simulink model "PMSM_traditional_SMO_PLL_Leon"  (R2024b)
settings: Solver=FixedStepAuto  StartTime=0.0  StopTime=0.5  FixedStep=1e-6  RelTol=1e-4  EnableMultiTasking=on
PreLoadFcn:
  | flux =0.0037
  | Ld =1.2050e-04
  | Lq =1.8000e-04
  | Pn =4
  | R =0.0830
  | Ts =5.0000e-05
undefined symbols (not defined in the file): DiscIntNeverNeededParam
libraries: mcbcontrolslib x3, simulink x2, powerlib_extras x2, spsDCVoltageSourceLib x1, spsPermanentMagnetSynchronousMachineLib x1, spsUniversalBridgeLib x1, spspowerguiLib x1
settings Model: LastModifiedBy=SESA504213
settings SolverCC: ZeroCrossControl=DisableAll  AlgebraicLoopSolver=TrustRegion  AutoInsertRateTranBlk=on
settings DataIOCC: LimitDataPoints=on  SaveFormat=Array  SignalLoggingSaveFormat=ModelDataLogs  ReturnWorkspaceOutputs=off
settings OptimizationCC: ReuseModelBlockBuffer=off  ExpressionDepthLimit=2147483647  InitFltsAndDblsToZero=on  LifeSpan=inf
settings DebuggingCC: UnderspecifiedInitializationDetection=Classic  MergeDetectMultiDrivingBlocksExec=none  SolverPrmCheckMsg=warning  FcnCallInpInsideContextMsg=warning  UnconnectedInputMsg=warning  UnconnectedOutputMsg=warning  UnconnectedLineMsg=warning  StateNameClashWarn=warning  SFUnexpectedBacktrackingDiag=warning  SFNoUnconditionalDefaultTransitionDiag=warning  SFExecutionAtInitializationDiag=none  ArithmeticOperatorsInVariantConditions=warning
settings HardwareCC: ProdBitPerPointer=32  ProdBitPerSizeT=32  ProdBitPerPtrDiffT=32  ProdLargestAtomicFloat=None  ProdIntDivRoundTo=Undefined  ProdEndianess=Unspecified  ProdWordSize=32  ProdHWDeviceType=32-bit Generic
settings ModelReferenceCC: EnableRefExpFcnMdlSchedulingChecks=on  PropagateSignalLabelsOutOfModel=off
settings SFSimCC: SimUseLocalCustomCode=off  CustomCodeUndefinedFunction=UseInterfaceOnly
settings RTWCC: RTWUseLocalCustomCode=off  GPUComputeCapability=3.5  DLArmComputeVersion=19.05
settings CodeAppCC: StateflowObjectComments=on
settings GRTTargetCC: TargetLangStandard=C89/C90 (ANSI)  CombineOutputUpdateFcns=off  GRTInterface=on
settings ConfigComp: CovMetricSettings=dw  CovSaveCumulativeToWorkspaceVar=on  CovSaveSingleToWorkspaceVar=on  CovExternalEMLEnable=off  CovSFcnEnable=off
settings SimscapeCC: SimscapeNormalizeSystem=off

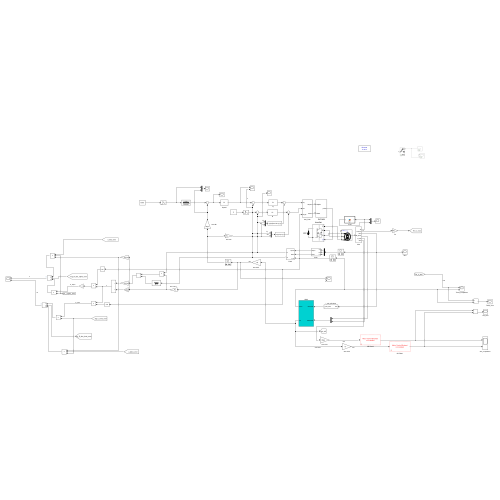
[thumbnail: Simulink's stored preview of the top-level diagram]
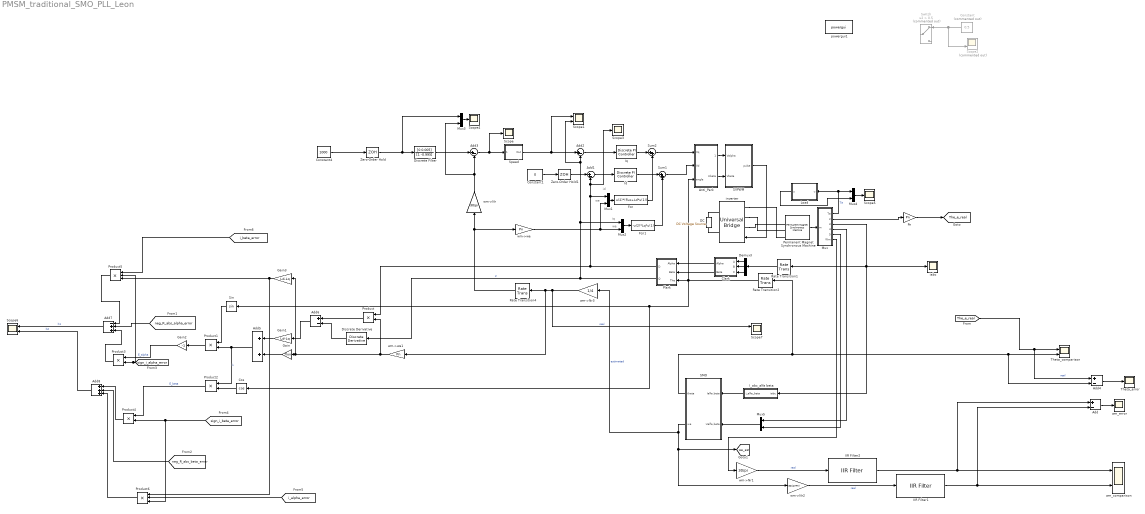
== system PMSM_traditional_SMO_PLL_Leon ==
  note: iq
  note: we
  note: we
  note: id
  Add : Sum  Inputs=+-
  Add1 : Sum  Inputs=|+-
  Add2 : Sum  Inputs=|+-
  Add3 : Sum  Inputs=|+-
  Add4 : Sum  Inputs=+-
  Add5 : Sum
  Add6 : Sum  Inputs=+-
  Add7 : Sum  Inputs=-++
  Add8 : Sum  Inputs=+++
  Anti_Park : Subsystem
  Clark : Subsystem
  Constant : Constant  Commented=on  Value=0.5
  Constant1 : Constant  Value=0
  Constant4 : Constant  Value=1000
  Cos : Trigonometry  Operator=cos
  DC : spsDCVoltageSourceLib/DC Voltage Source  Amplitude=24  Measurements=None
  Demux3 : Demux  Outputs=3
  Discrete Derivative : simulink/Discrete/Discrete Derivative  gainval=1.0  ICPrevScaledInput=0.0  OutMin=[]  OutMax=[]  OutDataType=fixdt(1, 16)  OutScaling=2^-10  DoSatur=off
  Discrete Filter : DiscreteFilter  Numerator=[0 0.005]  Denominator=[1 -0.995]  InitialStates=0.001
  Fcn : Fcn  Expr=u(2)*(flux+Ld*u(1))
  Fcn1 : Fcn  Expr=-u(2)*Lq*u(1)
  Gain : Gain  Gain=flux
  Gain1 : Gain  Gain=Ld-Lq
  Gain2 : Gain  Gain=-1
  Gain3 : Gain  Gain=Ld-Lq
  IIR Filter1 : mcbcontrolslib/IIR Filter  VariantControl=Low Pass Filter  VariantSelect=Low-pass  Filter_constant=0.0004  advancedSettings=on  Ts=1e-6  cutOff_freq=63.6875
  IIR Filter2 : mcbcontrolslib/IIR Filter  VariantControl=Low Pass Filter  VariantSelect=Low-pass  Filter_constant=0.0004  advancedSettings=on  Ts=1e-6  cutOff_freq=63.6875
  I_abc_alfa beta : Subsystem
  Id : powerlib_extras/Discrete  Control Blocks/Discrete PI Controller  Kp=Ld*4000/2  Ki=R*4000/2  Par_Limits=[24*0.9*sqrt(1/3) -24*0.9*sqrt(1/3)]  Init=0  Ts=Ts
  Iq : powerlib_extras/Discrete  Control Blocks/Discrete PI Controller  Kp=Lq*4000/2  Ki=R*4000/2  Par_Limits=[24*0.9*sqrt(1/3) -24*0.9*sqrt(1/3)]  Init=0  Ts=Ts
  Load : MATLAB Function  TreatAsAtomicUnit=on
  Mux : Subsystem
  Mux{1..5} (5 alike) : Mux  Inputs=2
  Permanent Magnet Synchronous Machine : spsPermanentMagnetSynchronousMachineLib/Permanent Magnet Synchronous Machine  NbPhases=3  FluxDistribution=Sinusoidal  RotorType=Salient-pole  MechanicalLoad=Torque Tm  PresetModel=No  ShowDetailedParameters=on  MeasurementBus=off  Resistance=R  Inductance=0  dqInductances=[Ld,Lq]  La=0.000835  MachineConstant=Flux linkage established by magnets (V.s)  Flux=flux  VoltageCst=2.6844  TorqueCst=0.0222  Flat=0  Mechanical=[1e-5,1e-5,Pn]  PolePairs=4  InitialConditions=[0,0,0,0]  InitialConditions5ph=[0 0 0 0 0 0]  RefAngle=Aligned with phase A axis (original Park)  IterativeDiscreteModel=Trapezoidal non iterative  TsBlock=-1  TsPowergui=0
      settings: AttributesFormatString=\n
  Plark : Subsystem
  Pn : Gain  Gain=Pn
  Product{,1..4} (5 alike) : Product
  Product5 : Product  Inputs=3
  Product6 : Product  Inputs=3
  Rate Transition1 : RateTransition  OutPortSampleTime=Ts
  Rate Transition2 : RateTransition  OutPortSampleTime=Ts
  Rate Transition4 : RateTransition  OutPortSampleTime=Ts
  SMO : Subsystem
  SVPWM : Subsystem
  Scope{,3..5} (4 alike) : Scope
  Scope1 : Scope  NumInputPorts=2
  Scope2 : Scope  Commented=on  NumInputPorts=2
  Scope6 : Scope  NumInputPorts=2
  Scope7 : Scope  NumInputPorts=2
  Sin : Trigonometry
  Speed : Subsystem  AncestorBlock=|  DialogController=POWERSYS.PowerSysDialog  mask(Discrete PI Controller){Kp=0.0453/2, Ki=1.1381/2, Par_Limits=[30 -30], Init=0, Ts=Ts}
      | powerlib_extras/Discrete 
      | Control Blocks/Discrete
      | PI Controller
      mask prompts: Kp "Proportional gain (Kp):"; Ki "Integral gain (Ki):"; Par_Limits "Output limits: [ Upper   Lower ]"; Init "Output initial value:"; Ts "Sample time:"
      mask help: This block implements a discrete PI controller.
      mask init:
      | UpperLimit=Par_Limits(1);
      | LowerLimit=Par_Limits(2);
      | power_initmask();
      mask Help: This block is part of a subset of blocks in the Extras library that does not have documentation associated with it, other than the block mask description.
      mask Display: disp('PI');
  Sum1 : Sum  Inputs=|++
  Sum2 : Sum  Inputs=|++
  Switch : Switch  Commented=on  Criteria=u2 > Threshold  Threshold=0.5  SaturateOnIntegerOverflow=off  InputSameDT=off
  Theta_comparison : Scope  NumInputPorts=2
  Theta_error : Scope
  Zero-Order Hold : ZeroOrderHold  SampleTime=Ts
  Zero-Order Hold1 : ZeroOrderHold  SampleTime=Ts
  iabc : Scope
  inverter : spsUniversalBridgeLib/Universal Bridge  Arms=3  SnubberResistance=100  SnubberCapacitance=1e-5  Device=MOSFET / Diodes  Ron=1e-3  Lon=0  ForwardVoltages="[  0  0  ]"  ForwardVoltage=0  GTOparameters=[ 10e-6 , 20e-6 ]  IGBTparameters=[ 1e-6 , 2e-6 ]  Measurements=None  Measurements_2=None  converterType=Rectifier
  powergui1 : spspowerguiLib/powergui  Priority=1  SimulationMode=Discrete  SampleTime=1e-6  frequency=60  Iterations=50  frequencyindice=0  Pbase=100e6  ErrMax=1e-4  UnitsV=kV  UnitsW=MW  buscounter=0  FunctionMessages=off  echomessages=off  EnableUseOfTLC=off  CurrentSourceSwitches=off  DisableSnubberDevices=off  DisableRonSwitches=off  DisableVfSwitches=off  DisplayEquations=off  AutomaticDiscreteSolvers=off  SolverType=Tustin/Backward Euler (TBE)  Interpol=off  ExternalGateDelay=off  methode=off  Ts=100  x0status=blocks  SPID=on  SwTol=0  HookPort=off  NonlinearTolerance=1e-4  nMaxIteration=100  ContinueOnMaxIteration=off  RestoreLinks=warning  ResistiveCurrentMeasurement=off  Frange=[0:2:500]  Ylog=off  Xlog=on  ShowGrid=off  save=off  variable=ZData  structure=0  ZoomFFT=off  StartTime=0.0  cycles=1  DisplayStyle=1  fundamental=60  FreqAxis=off  MaxFrequency=1000  frequencyindicesteady=1  RmsSteady=1  display=off
  wm->Nr : Gain  Gain=30/pi
  wm->Nr1 : Gain  Gain=30/pi
  wm->Nr2 : Gain  Gain=30/(pi*Pn)
  wm->Nr3 : Gain  Gain=1/4
  wm->we : Gain  Gain=Pn
  wm->we1 : Gain  Gain=Pn
  wm_comparison : Scope  NumInputPorts=2
  wm_error : Scope
  tag scope: The_e_real=global, we_est=global
  wires:
  Permanent Magnet Synchronous Machine/1 -> Mux/1(m)
  Add3/1 -> Speed/1(Error), Scope/1
  Fcn/1 -> Sum2/2
  Fcn1/1 -> Sum1/2
  Add1/1 -> Id/1
  wm->Nr/1 -> Mux3/2, Add3/2
  Id/1 -> Sum1/1
  wm->we/1 -> Mux2/2, Mux1/2
  Mux1/1 -> Fcn/1
  Mux2/1 -> Fcn1/1
  Add2/1 -> Iq/1
  Iq/1 -> Sum2/1
  Sum2/1 -> Anti_Park/1(Vq)
  Sum1/1 -> Anti_Park/2(Vd)
  Mux/2(Thetam) -> Pn/1
  SVPWM/1(pulse) -> inverter/1
  Anti_Park/1(Ualpha) -> SVPWM/1(Valpha)
  Anti_Park/2(Ubeta) -> SVPWM/2(Vbeta)
  Clark/1(Alpha) -> Plark/1(Alpha)
  Demux3/1 -> Clark/1(A)
  Demux3/2 -> Clark/2(B)
  Demux3/3 -> Clark/3(C)
  Clark/2(Beta) -> Plark/2(Beta)
  Plark/2(Q) -> Discrete Derivative/1, Mux2/1, Scope1/2, Add2/2  "2"
  Constant/1 -> Scope2/2, Switch/1
  Speed/1(Out) -> Scope1/1, Add2/1
  Mux/3(Iabc) -> I_abc_alfa beta/1(iabc), Rate Transition1/1, iabc/1
  Pn/1 -> [The_e_real]
  Plark/1(D) -> Product/1, Mux1/1, Scope3/1, Add1/2
  Rate Transition4/1 -> wm->Nr/1, wm->we/1
  Constant4/1 -> Zero-Order Hold/1
  Constant1/1 -> Zero-Order Hold1/1
  Zero-Order Hold1/1 -> Add1/1
  Rate Transition1/1 -> Demux3/1
  Rate Transition2/1 -> Cos/1, Sin/1, Anti_Park/3(angle), Plark/3(The)
  Zero-Order Hold/1 -> Mux3/1, Discrete Filter/1
  Discrete Filter/1 -> Add3/1
  Mux3/1 -> Scope4/1
  Load/1(y) -> Mux4/2
  Mux/1(Te) -> Mux4/1, Load/1(u)  "Te"
  Mux4/1 -> Scope5/1
  I_abc_alfa beta/1(i_alfa_beta) -> SMO/1(Ialfa,beta)
  Mux5/1 -> SMO/2(Ualfa,beta)
  SMO/1(theta) -> Rate Transition2/1, Add4/2, Theta_comparison/2
  wm->Nr1/1 -> IIR Filter2/1  "real"
  SMO/2(we) -> wm->Nr3/1, wm->Nr2/1, [we_est]  "estimated"
  [The_e_real] -> Add4/1, Theta_comparison/1  "real"
  Add/1 -> wm_error/1
  Add4/1 -> Theta_error/1
  Mux/4(u_alpha) -> Mux5/1
  Mux/5(u_beta) -> Mux5/2
  wm->Nr2/1 -> IIR Filter1/1  "real"
  wm->we1/1 -> Gain3/1, Gain/1, Product/2
  Gain/1 -> Add5/2
  Gain1/1 -> Add5/1
  Product/1 -> Add6/1
  Discrete Derivative/1 -> Add6/2
  Add6/1 -> Gain1/1
  Add5/1 -> Product2/1, Product1/2  "k"
  Sin/1 -> Product1/1
  Product1/1 -> Gain2/1
  Gain2/1 -> Product3/1  "E_alpha"
  Cos/1 -> Product2/2
  Product2/1 -> Product4/1  "E_beta"
  [neg_R_abs_beta_error] -> Add8/2
  Add7/1 -> Scope6/1  "h1"
  Add8/1 -> Scope6/2  "h2"
  [sign_i_alpha_error] -> Product3/2, Product5/2
  Product4/1 -> Add8/1
  [sign_i_beta_error] -> Product6/3, Product4/2
  Product3/1 -> Add7/3
  [neg_R_abs_alpha_error] -> Add7/2
  Gain3/1 -> Product5/3, Product6/1
  [i_beta_error] -> Product5/1
  Product5/1 -> Add7/1
  Product6/1 -> Add8/3
  [i_alpha_error] -> Product6/2
  IIR Filter1/1 -> Add/2, wm_comparison/2
  IIR Filter2/1 -> Add/1, wm_comparison/1
  wm->Nr3/1 -> Scope7/1, wm->we1/1, Rate Transition4/1  "real"
  Mux/6(Wm) -> wm->Nr1/1
  connections:
  DC/RConn1 -- inverter/RConn1
  DC/LConn1 -- inverter/RConn2
  inverter/LConn1 -- Permanent Magnet Synchronous Machine/LConn1
  inverter/LConn2 -- Permanent Magnet Synchronous Machine/LConn2
  inverter/LConn3 -- Permanent Magnet Synchronous Machine/LConn3

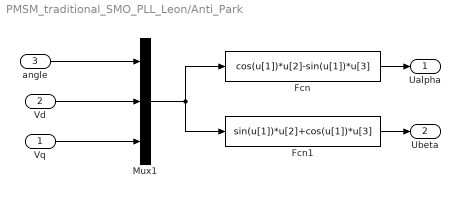
== system PMSM_traditional_SMO_PLL_Leon/Anti_Park ==
  Vq : Inport
  Vd : Inport  Port=2
  angle : Inport  Port=3
  Fcn : Fcn  Expr=cos(u[1])*u[2]-sin(u[1])*u[3]
  Fcn1 : Fcn  Expr=sin(u[1])*u[2]+cos(u[1])*u[3]
  Mux1 : Mux  Inputs=3
  Ualpha : Outport
  Ubeta : Outport  Port=2
  wires:
  Fcn1/1 -> Ubeta/1
  Fcn/1 -> Ualpha/1
  Mux1/1 -> Fcn/1, Fcn1/1
  Vd/1 -> Mux1/2
  Vq/1 -> Mux1/3
  angle/1 -> Mux1/1

== system PMSM_traditional_SMO_PLL_Leon/Clark ==
  A : Inport
  B : Inport  Port=2
  C : Inport  Port=3
  Mux : Mux  Inputs=3
  alpha : Fcn  Expr=(u(1)-0.5*(u(2)+u(3)))*2/3
  beta : Fcn  Expr=sqrt(3)/2*(u(2)-u(3))*2/3
  Alpha : Outport
  Beta : Outport  Port=2
  wires:
  alpha/1 -> Alpha/1
  B/1 -> Mux/2
  C/1 -> Mux/3
  A/1 -> Mux/1
  Mux/1 -> beta/1, alpha/1
  beta/1 -> Beta/1

== system PMSM_traditional_SMO_PLL_Leon/I_abc_alfa beta ==
  iabc : Inport
  Fcn : Fcn  Expr=(2*u(1)-u(2)-u(3))/3
  Fcn1 : Fcn  Expr=(u(2)-u(3))/(3^(1/2))
  Mux2 : Mux  Inputs=2
  i_alfa_beta : Outport
  wires:
  iabc/1 -> Fcn/1, Fcn1/1
  Mux2/1 -> i_alfa_beta/1
  Fcn/1 -> Mux2/1
  Fcn1/1 -> Mux2/2

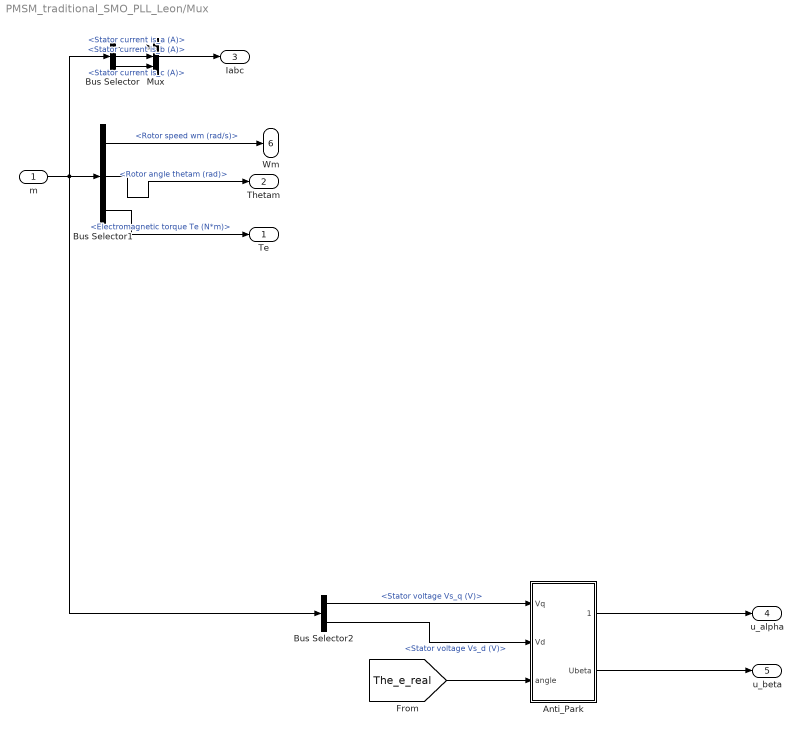
== system PMSM_traditional_SMO_PLL_Leon/Mux ==
  m : Inport
  Anti_Park : Subsystem
  Bus Selector : BusSelector  OutputSignals=Stator current is_a (A),Stator current is_b (A),Stator current is_c (A)
  Bus Selector1 : BusSelector  OutputSignals=Rotor speed wm (rad/s),Rotor angle thetam (rad),Electromagnetic torque Te (N*m)
  Bus Selector2 : BusSelector  OutputSignals=Stator voltage Vs_q (V),Stator voltage Vs_d (V)
  Mux : Mux  Inputs=3
  Te : Outport
  Thetam : Outport  Port=2
  Iabc : Outport  Port=3
  u_alpha : Outport  Port=4
  u_beta : Outport  Port=5
  Wm : Outport  Port=6
  wires:
  Bus Selector1/1 -> Wm/1  "<Rotor speed wm (rad/s)>"
  Bus Selector1/2 -> Thetam/1  "<Rotor angle thetam (rad)>"
  Bus Selector1/3 -> Te/1  "<Electromagnetic torque Te (N*m)>"
  m/1 -> Bus Selector2/1, Bus Selector/1, Bus Selector1/1
  Bus Selector/2 -> Mux/2  "<Stator current is_b (A)>"
  Bus Selector/3 -> Mux/3  "<Stator current is_c (A)>"
  Bus Selector/1 -> Mux/1  "<Stator current is_a (A)>"
  Mux/1 -> Iabc/1
  Bus Selector2/2 -> Anti_Park/2(Vd)  "<Stator voltage Vs_d (V)>"
  Bus Selector2/1 -> Anti_Park/1(Vq)  "<Stator voltage Vs_q (V)>"
  Anti_Park/1(Ualpha) -> u_alpha/1
  [The_e_real] -> Anti_Park/3(angle)
  Anti_Park/2(Ubeta) -> u_beta/1

== system PMSM_traditional_SMO_PLL_Leon/Plark ==
  Alpha : Inport
  Beta : Inport  Port=2
  The : Inport  Port=3
  Mux : Mux  Inputs=3
  d : Fcn  Expr=u(1)*cos(u(3))+u(2)*sin(u(3))
  q : Fcn  Expr=-u(1)*sin(u(3))+u(2)*cos(u(3))
  D : Outport
  Q : Outport  Port=2
  wires:
  d/1 -> D/1
  Beta/1 -> Mux/2
  Alpha/1 -> Mux/1
  Mux/1 -> q/1, d/1
  q/1 -> Q/1
  The/1 -> Mux/3

== system PMSM_traditional_SMO_PLL_Leon/SMO ==
  Ialfa,beta : Inport
  Ualfa,beta : Inport  Port=2
  PLL : Subsystem
  SMO : Subsystem
  theta : Outport
  we : Outport  Port=2
  wires:
  Ualfa,beta/1 -> SMO/1(Ualfa,beta)
  Ialfa,beta/1 -> SMO/2(Ialfa,beta)
  SMO/1(Ealpha^) -> PLL/1(e_alpha_est)
  SMO/2(Ebeta^) -> PLL/2(e_beta_est)
  PLL/1(theta_est) -> theta/1
  PLL/2(we_est) -> we/1

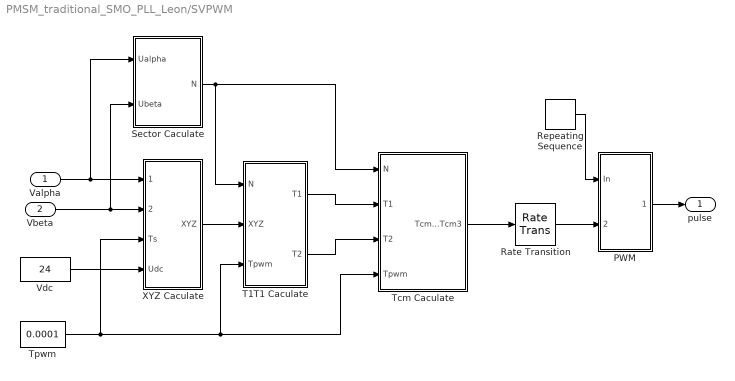
== system PMSM_traditional_SMO_PLL_Leon/SVPWM ==
  Valpha : Inport
  Vbeta : Inport  Port=2
  PWM : Subsystem
  Rate Transition : RateTransition  OutPortSampleTime=1e-6
  Repeating Sequence : simulink/Sources/Repeating Sequence  rep_seq_t=[0 0.00005 0.0001]  rep_seq_y=[0 0.00005 0]
  Sector Caculate : Subsystem
  T1T1 Caculate : Subsystem
  Tcm Caculate : Subsystem
  Tpwm : Constant  Value=0.0001
  Vdc : Constant  Value=24
  XYZ Caculate : Subsystem
  pulse : Outport
  wires:
  PWM/1(PWM) -> pulse/1
  Repeating Sequence/1 -> PWM/1(In)
  Vbeta/1 -> XYZ Caculate/2(Ubeta), Sector Caculate/2(Ubeta)
  T1T1 Caculate/1(T1) -> Tcm Caculate/2(T1)
  Valpha/1 -> XYZ Caculate/1(Ualpha), Sector Caculate/1(Ualpha)
  T1T1 Caculate/2(T2) -> Tcm Caculate/3(T2)
  Sector Caculate/1("N ") -> Tcm Caculate/1(N), T1T1 Caculate/1(N)
  XYZ Caculate/1(XYZ) -> T1T1 Caculate/2(XYZ)
  Tpwm/1 -> XYZ Caculate/3(Ts), Tcm Caculate/4(Tpwm), T1T1 Caculate/3(Tpwm)
  Vdc/1 -> XYZ Caculate/4(Udc)
  Tcm Caculate/1(Tcm1 Tcm2 Tcm3) -> Rate Transition/1
  Rate Transition/1 -> PWM/2(Tcm123)

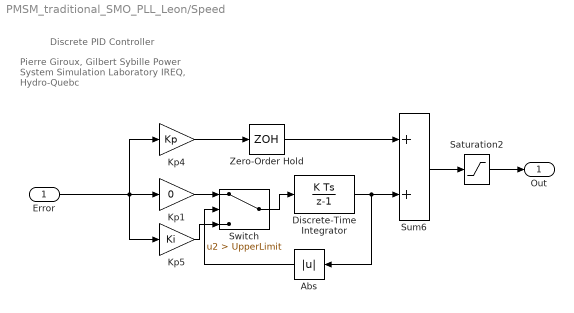
== system PMSM_traditional_SMO_PLL_Leon/Speed ==
  note: Discrete PID Controller
  note: Pierre Giroux, Gilbert Sybille
      | Power System Simulation Laboratory
      | IREQ, Hydro-Quebc
  Error : Inport  SampleTime=Ts
  Abs : Abs  SaturateOnIntegerOverflow=off
  Discrete-Time Integrator : DiscreteIntegrator  InitialCondition=Init  SampleTime=Ts  LimitOutput=on  UpperSaturationLimit=UpperLimit  LowerSaturationLimit=LowerLimit  ICPrevOutput=DiscIntNeverNeededParam  ICPrevScaledInput=DiscIntNeverNeededParam
  Kp1 : Gain  Gain=0  SaturateOnIntegerOverflow=on  SampleTime=Ts  OutDataTypeStr=Inherit: Same as input  ParamDataTypeStr=Inherit: Same as input
  Kp4 : Gain  Gain=Kp  SaturateOnIntegerOverflow=on  SampleTime=Ts  OutDataTypeStr=Inherit: Same as input  ParamDataTypeStr=Inherit: Same as input
  Kp5 : Gain  Gain=Ki  SaturateOnIntegerOverflow=on  SampleTime=Ts  OutDataTypeStr=Inherit: Same as input  ParamDataTypeStr=Inherit: Same as input
  Saturation2 : Saturate  UpperLimit=UpperLimit  LowerLimit=LowerLimit  SampleTime=Ts
  Sum6 : Sum  InputSameDT=on  SaturateOnIntegerOverflow=on  SampleTime=Ts  OutDataTypeStr=Inherit: Same as first input
  Switch : Switch  Criteria=u2 > Threshold  Threshold=UpperLimit  SaturateOnIntegerOverflow=off  InputSameDT=off
  Zero-Order Hold : ZeroOrderHold  SampleTime=Ts
  Out : Outport  SampleTime=Ts  InitialOutput=0  VectorParamsAs1DForOutWhenUnconnected=off
  wires:
  Zero-Order Hold/1 -> Sum6/1
  Saturation2/1 -> Out/1
  Discrete-Time Integrator/1 -> Abs/1, Sum6/2
  Kp4/1 -> Zero-Order Hold/1
  Sum6/1 -> Saturation2/1
  Error/1 -> Kp4/1, Kp1/1, Kp5/1
  Switch/1 -> Discrete-Time Integrator/1
  Abs/1 -> Switch/2
  Kp5/1 -> Switch/3
  Kp1/1 -> Switch/1

== system PMSM_traditional_SMO_PLL_Leon/Mux/Anti_Park ==
  Vq : Inport
  Vd : Inport  Port=2
  angle : Inport  Port=3
  Fcn : Fcn  Expr=cos(u[1])*u[2]-sin(u[1])*u[3]
  Fcn1 : Fcn  Expr=sin(u[1])*u[2]+cos(u[1])*u[3]
  Mux1 : Mux  Inputs=3
  Ualpha : Outport
  Ubeta : Outport  Port=2
  wires:
  Fcn1/1 -> Ubeta/1
  Fcn/1 -> Ualpha/1
  Mux1/1 -> Fcn/1, Fcn1/1
  Vd/1 -> Mux1/2
  Vq/1 -> Mux1/3
  angle/1 -> Mux1/1

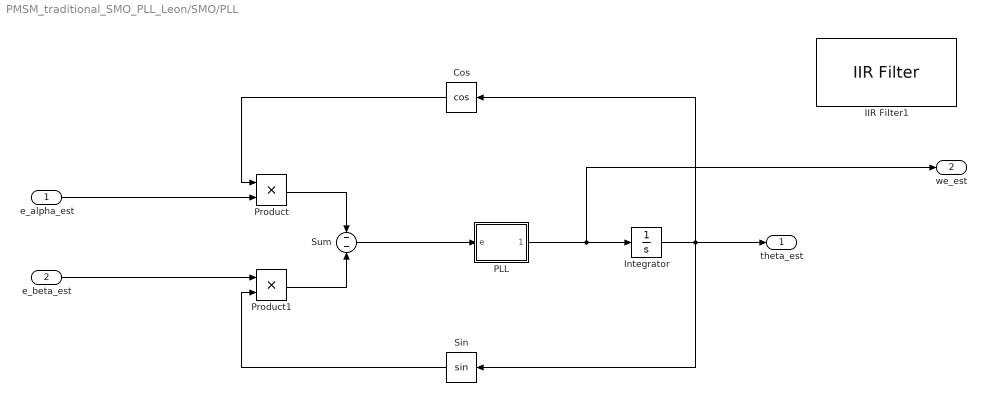
== system PMSM_traditional_SMO_PLL_Leon/SMO/PLL ==
  e_alpha_est : Inport
  e_beta_est : Inport  Port=2
  Cos : Trigonometry  Operator=cos
  IIR Filter1 : mcbcontrolslib/IIR Filter  VariantControl=Low Pass Filter  VariantSelect=Low-pass  Filter_constant=0.0004  advancedSettings=on  Ts=1e-6  cutOff_freq=63.6875
  Integrator : Integrator
  PLL : Subsystem
      mask Display: disp('PI')
  Product : Product
  Product1 : Product
  Sin : Trigonometry
  Sum : Sum  Inputs=--
  theta_est : Outport
  we_est : Outport  Port=2
  wires:
  e_alpha_est/1 -> Product/2
  Cos/1 -> Product/1
  Product/1 -> Sum/1
  e_beta_est/1 -> Product1/1
  Product1/1 -> Sum/2
  Sin/1 -> Product1/2
  Integrator/1 -> Cos/1, theta_est/1, Sin/1
  Sum/1 -> PLL/1(e)
  PLL/1(output) -> we_est/1, Integrator/1

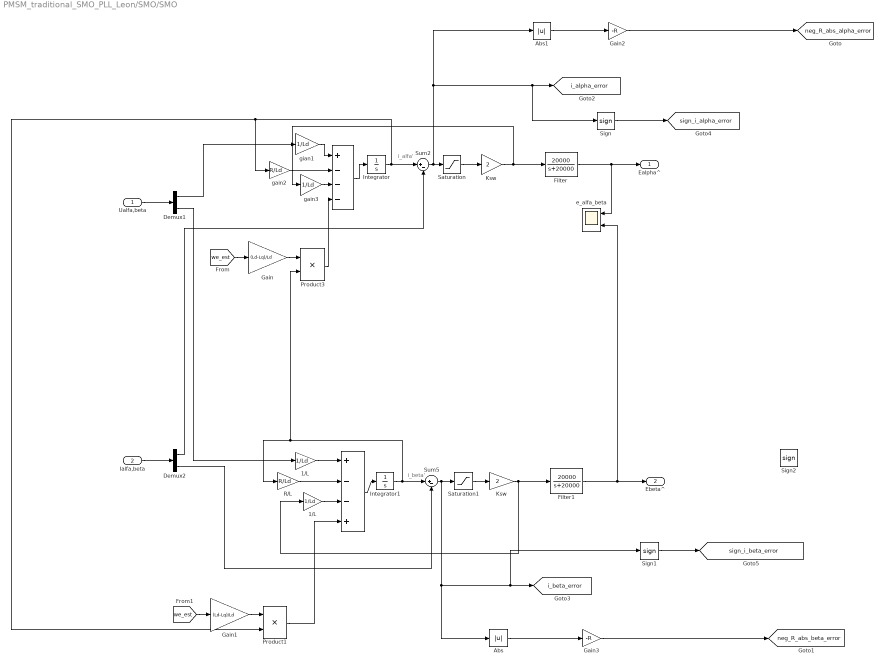
== system PMSM_traditional_SMO_PLL_Leon/SMO/SMO ==
  note: i_alfa'
  note: i_beta'
  Ualfa,beta : Inport
  Ialfa,beta : Inport  Port=2
  " " : Sum  Inputs=+---
  "   " : Sum  Inputs=+--+
  " 1/L" : Gain  Gain=1/Ld
  " 1/L " : Gain  Gain=1/Ld
  Abs : Abs  SaturateOnIntegerOverflow=off
  Abs1 : Abs  SaturateOnIntegerOverflow=off
  Demux1 : Demux  Outputs=2
  Demux2 : Demux  Outputs=2
  Filter : TransferFcn  Numerator=[20000]  Denominator=[1 20000]
  Filter1 : TransferFcn  Numerator=[20000]  Denominator=[1 20000]
  Gain : Gain  Gain=(Ld-Lq)/Ld
  Gain1 : Gain  Gain=(Ld-Lq)/Ld
  Gain2 : Gain  Gain=-R
  Gain3 : Gain  Gain=-R
  Integrator : Integrator
  Integrator1 : Integrator
  Ksw : Gain  Gain=2
  "Ksw " : Gain  Gain=2
  Product1 : Product  RndMeth=Zero
  Product3 : Product  RndMeth=Zero
  "R/L " : Gain  Gain=R/Ld
  Saturation : Saturate  UpperLimit=1  LowerLimit=-1
  Saturation1 : Saturate  UpperLimit=1  LowerLimit=-1
  Sign : Signum  ZeroCross=off
  Sign1 : Signum  ZeroCross=off
  Sign2 : Signum  ZeroCross=off
  Sum2 : Sum  Inputs=|+-
  Sum5 : Sum  Inputs=|+-
  e_alfa_beta : Scope  NumInputPorts=2
  gain2 : Gain  Gain=R/Ld
  gain3 : Gain  Gain=1/Ld
  gian1 : Gain  Gain=1/Ld
  Ealpha^ : Outport
  Ebeta^ : Outport  Port=2
  tag scope: i_alpha_error=global, i_beta_error=global, neg_R_abs_alpha_error=global, neg_R_abs_beta_error=global, sign_i_alpha_error=global, sign_i_beta_error=global
  wires:
  Integrator/1 -> Sum2/1, Product1/2, gain2/1
  Saturation/1 -> Ksw/1
  Ksw/1 -> gain3/1, Filter/1
  Integrator1/1 -> Sum5/1, Product3/2, "R/L "/1
  Sum5/1 -> Saturation1/1, Abs/1, Sign1/1, [i_beta_error]
  Saturation1/1 -> "Ksw "/1
  "Ksw "/1 -> " 1/L "/1, Filter1/1
  Demux2/1 -> Sum2/2
  Demux2/2 -> Sum5/2
  gian1/1 -> " "/1
  gain2/1 -> " "/2
  gain3/1 -> " "/3
  " "/1 -> Integrator/1
  Demux1/2 -> " 1/L"/1
  " 1/L"/1 -> "   "/1
  "R/L "/1 -> "   "/2
  "   "/1 -> Integrator1/1
  " 1/L "/1 -> "   "/3
  Sum2/1 -> Sign/1, [i_alpha_error], Abs1/1, Saturation/1
  Filter1/1 -> e_alfa_beta/2, Ebeta^/1
  Filter/1 -> Ealpha^/1, e_alfa_beta/1
  Demux1/1 -> gian1/1
  Ialfa,beta/1 -> Demux2/1
  Ualfa,beta/1 -> Demux1/1
  [we_est] -> Gain/1
  Gain/1 -> Product3/1
  Product3/1 -> " "/4
  Gain1/1 -> Product1/1
  [we_est] -> Gain1/1
  Product1/1 -> "   "/4
  Gain2/1 -> [neg_R_abs_alpha_error]
  Gain3/1 -> [neg_R_abs_beta_error]
  Abs/1 -> Gain3/1
  Abs1/1 -> Gain2/1
  Sign/1 -> [sign_i_alpha_error]
  Sign1/1 -> [sign_i_beta_error]

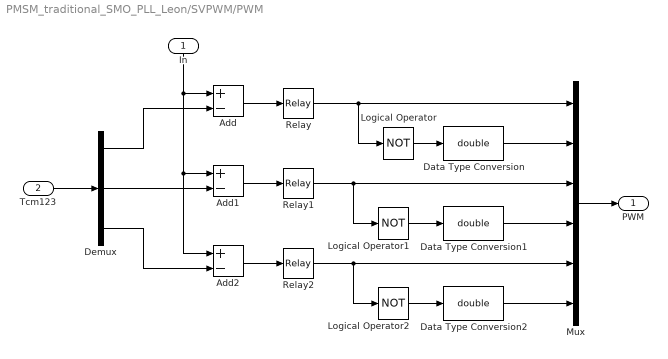
== system PMSM_traditional_SMO_PLL_Leon/SVPWM/PWM ==
  In : Inport
  Tcm123 : Inport  Port=2
  Add : Sum  Inputs=+-
  Add1 : Sum  Inputs=+-
  Add2 : Sum  Inputs=+-
  Data Type Conversion : DataTypeConversion  OutDataTypeStr=double  SaturateOnIntegerOverflow=off  RndMeth=Floor
  Data Type Conversion1 : DataTypeConversion  OutDataTypeStr=double  SaturateOnIntegerOverflow=off  RndMeth=Floor
  Data Type Conversion2 : DataTypeConversion  OutDataTypeStr=double  SaturateOnIntegerOverflow=off  RndMeth=Floor
  Demux : Demux  Outputs=3
  Logical Operator : Logic  Operator=NOT  AllPortsSameDT=off  OutDataTypeStr=boolean
  Logical Operator1 : Logic  Operator=NOT  AllPortsSameDT=off  OutDataTypeStr=boolean
  Logical Operator2 : Logic  Operator=NOT  AllPortsSameDT=off  OutDataTypeStr=boolean
  Mux : Mux  Inputs=6
  Relay : Relay  OffSwitchValue=-eps
  Relay1 : Relay  OffSwitchValue=-eps
  Relay2 : Relay  OffSwitchValue=-eps
  PWM : Outport
  wires:
  Demux/3 -> Add2/2
  Demux/2 -> Add1/2
  Demux/1 -> Add/2
  Relay2/1 -> Mux/5, Logical Operator2/1
  Relay1/1 -> Mux/3, Logical Operator1/1
  Relay/1 -> Logical Operator/1, Mux/1
  Mux/1 -> PWM/1
  Data Type Conversion/1 -> Mux/2
  Data Type Conversion1/1 -> Mux/4
  Data Type Conversion2/1 -> Mux/6
  Logical Operator2/1 -> Data Type Conversion2/1
  Logical Operator1/1 -> Data Type Conversion1/1
  Logical Operator/1 -> Data Type Conversion/1
  Add1/1 -> Relay1/1
  Add2/1 -> Relay2/1
  Add/1 -> Relay/1
  In/1 -> Add/1, Add2/1, Add1/1
  Tcm123/1 -> Demux/1

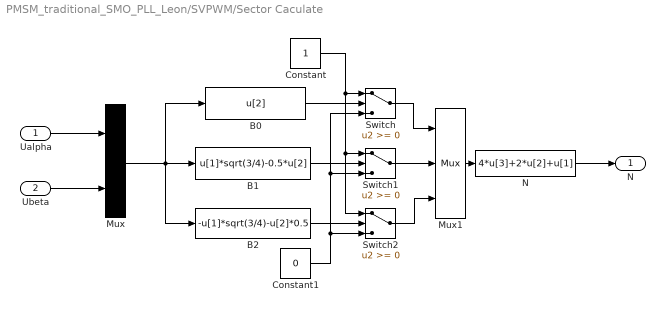
== system PMSM_traditional_SMO_PLL_Leon/SVPWM/Sector Caculate ==
  Ualpha : Inport
  Ubeta : Inport  Port=2
  B0 : Fcn  Expr=u[2]
  B1 : Fcn  Expr=u[1]*sqrt(3/4)-0.5*u[2]
  B2 : Fcn  Expr=-u[1]*sqrt(3/4)-u[2]*0.5
  Constant : Constant
  Constant1 : Constant  Value=0
  Mux : Mux  Inputs=2
  Mux1 : Mux  Inputs=3
  N : Fcn  Expr=4*u[3]+2*u[2]+u[1]
  Switch : Switch  SaturateOnIntegerOverflow=off  InputSameDT=off
  Switch1 : Switch  SaturateOnIntegerOverflow=off  InputSameDT=off
  Switch2 : Switch  SaturateOnIntegerOverflow=off  InputSameDT=off
  "N " : Outport
  wires:
  Switch2/1 -> Mux1/3
  Switch/1 -> Mux1/1
  Ualpha/1 -> Mux/1
  Ubeta/1 -> Mux/2
  Mux/1 -> B2/1, B1/1, B0/1
  B0/1 -> Switch/2
  B1/1 -> Switch1/2
  B2/1 -> Switch2/2
  Constant/1 -> Switch/1, Switch2/1, Switch1/1
  Constant1/1 -> Switch/3, Switch1/3, Switch2/3
  Switch1/1 -> Mux1/2
  Mux1/1 -> N/1
  N/1 -> "N "/1

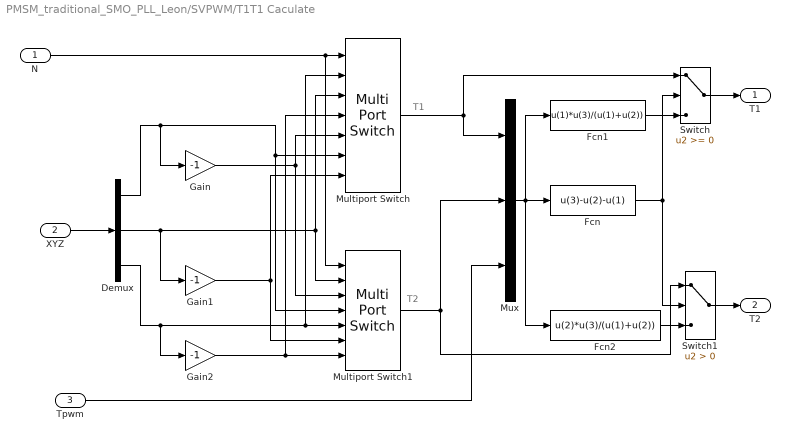
== system PMSM_traditional_SMO_PLL_Leon/SVPWM/T1T1 Caculate ==
  note: T1
  note: T2
  N : Inport
  XYZ : Inport  Port=2
  Tpwm : Inport  Port=3
  Demux : Demux  Outputs=3
  Fcn : Fcn  Expr=u(3)-u(2)-u(1)
  Fcn1 : Fcn  Expr=u(1)*u(3)/(u(1)+u(2))
  Fcn2 : Fcn  Expr=u(2)*u(3)/(u(1)+u(2))
  Gain : Gain  Gain=-1
  Gain1 : Gain  Gain=-1
  Gain2 : Gain  Gain=-1
  Multiport Switch : MultiPortSwitch  Inputs=6  SaturateOnIntegerOverflow=off  InputSameDT=off
  Multiport Switch1 : MultiPortSwitch  Inputs=6  SaturateOnIntegerOverflow=off  InputSameDT=off
  Mux : Mux  Inputs=3
  Switch : Switch  SaturateOnIntegerOverflow=off  InputSameDT=off
  Switch1 : Switch  Criteria=u2 > Threshold  SaturateOnIntegerOverflow=off  InputSameDT=off
  T1 : Outport
  T2 : Outport  Port=2
  wires:
  Tpwm/1 -> Mux/3
  XYZ/1 -> Demux/1
  Switch1/1 -> T2/1
  Switch/1 -> T1/1
  Fcn2/1 -> Switch1/3
  Fcn1/1 -> Switch/3
  Fcn/1 -> Switch/2, Switch1/2
  Mux/1 -> Fcn1/1, Fcn/1, Fcn2/1
  Multiport Switch/1 -> Switch/1, Mux/1
  Multiport Switch1/1 -> Switch1/1, Mux/2
  N/1 -> Multiport Switch/1, Multiport Switch1/1
  Demux/2 -> Multiport Switch/3, Multiport Switch1/2, Gain1/1
  Demux/3 -> Multiport Switch1/5, Multiport Switch/2, Gain2/1
  Demux/1 -> Multiport Switch/6, Multiport Switch1/4, Gain/1
  Gain/1 -> Multiport Switch1/3, Multiport Switch/5
  Gain2/1 -> Multiport Switch/4, Multiport Switch1/7
  Gain1/1 -> Multiport Switch1/6, Multiport Switch/7

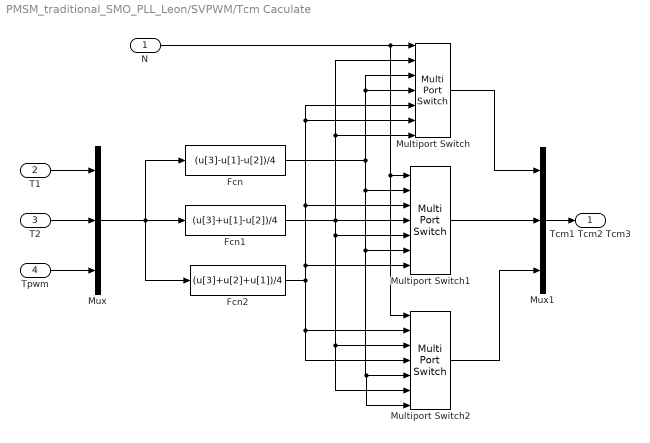
== system PMSM_traditional_SMO_PLL_Leon/SVPWM/Tcm Caculate ==
  N : Inport
  T1 : Inport  Port=2
  T2 : Inport  Port=3
  Tpwm : Inport  Port=4
  Fcn : Fcn  Expr=(u[3]-u[1]-u[2])/4
  Fcn1 : Fcn  Expr=(u[3]+u[1]-u[2])/4
  Fcn2 : Fcn  Expr=(u[3]+u[2]+u[1])/4
  Multiport Switch : MultiPortSwitch  Inputs=6  SaturateOnIntegerOverflow=off  InputSameDT=off
  Multiport Switch1 : MultiPortSwitch  Inputs=6  SaturateOnIntegerOverflow=off  InputSameDT=off
  Multiport Switch2 : MultiPortSwitch  Inputs=6  SaturateOnIntegerOverflow=off  InputSameDT=off
  Mux : Mux  Inputs=3
  Mux1 : Mux  Inputs=3
  Tcm1 Tcm2 Tcm3 : Outport
  wires:
  Mux/1 -> Fcn2/1, Fcn/1, Fcn1/1
  Tpwm/1 -> Mux/3
  T2/1 -> Mux/2
  T1/1 -> Mux/1
  Multiport Switch2/1 -> Mux1/3
  Multiport Switch1/1 -> Mux1/2
  Multiport Switch/1 -> Mux1/1
  Mux1/1 -> Tcm1 Tcm2 Tcm3/1
  Fcn/1 -> Multiport Switch/3, Multiport Switch/4, Multiport Switch1/6, Multiport Switch2/5, Multiport Switch2/7, Multiport Switch1/2
  Fcn1/1 -> Multiport Switch1/5, Multiport Switch2/3, Multiport Switch2/6, Multiport Switch1/4, Multiport Switch/7, Multiport Switch/2
  Fcn2/1 -> Multiport Switch/5, Multiport Switch/6, Multiport Switch1/3, Multiport Switch1/7, Multiport Switch2/2, Multiport Switch2/4
  N/1 -> Multiport Switch2/1, Multiport Switch1/1, Multiport Switch/1

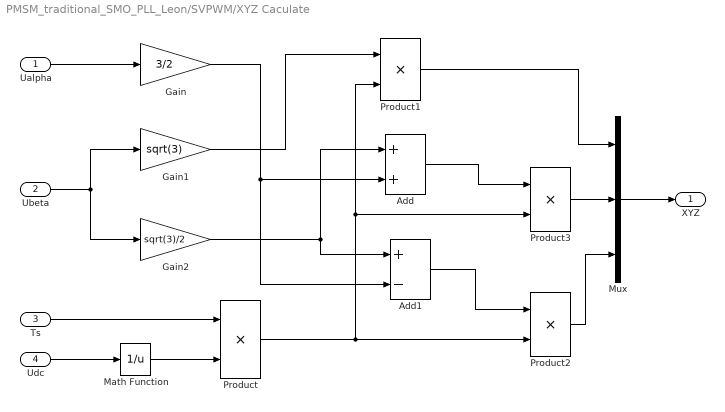
== system PMSM_traditional_SMO_PLL_Leon/SVPWM/XYZ Caculate ==
  Ualpha : Inport
  Ubeta : Inport  Port=2
  Ts : Inport  Port=3
  Udc : Inport  Port=4
  Add : Sum
  Add1 : Sum  Inputs=+-
  Gain : Gain  Gain=3/2
  Gain1 : Gain  Gain=sqrt(3)
  Gain2 : Gain  Gain=sqrt(3)/2
  Math Function : Math  Operator=reciprocal  SignedPower=on
  Mux : Mux  Inputs=3
  Product{,1..3} (4 alike) : Product  RndMeth=Zero
  XYZ : Outport
  wires:
  Mux/1 -> XYZ/1
  Product1/1 -> Mux/1
  Product3/1 -> Mux/2
  Product2/1 -> Mux/3
  Ualpha/1 -> Gain/1
  Ubeta/1 -> Gain2/1, Gain1/1
  Udc/1 -> Math Function/1
  Math Function/1 -> Product/2
  Ts/1 -> Product/1
  Gain1/1 -> Product1/1
  Product/1 -> Product2/2, Product1/2, Product3/2
  Gain/1 -> Add1/2, Add/2
  Gain2/1 -> Add/1, Add1/1
  Add1/1 -> Product2/1
  Add/1 -> Product3/1

== system PMSM_traditional_SMO_PLL_Leon/SMO/PLL/PLL ==
  e : Inport
  Add : Sum
  Integrator : Integrator
  Ki : Gain  Gain=36000
  Kp : Gain  Gain=540
  Saturation : Saturate  UpperLimit=1000  LowerLimit=-1000
  output : Outport
  wires:
  Ki/1 -> Integrator/1
  e/1 -> Kp/1, Ki/1
  Saturation/1 -> output/1
  Integrator/1 -> Add/2
  Kp/1 -> Add/1
  Add/1 -> Saturation/1

== matlab function PMSM_traditional_SMO_PLL_Leon/Load ==
  data: u input; y output
function y = fcn(u)

Ts=1e-6;
persistent  t k

if isempty(t)
    t=0;
end

if isempty(k)
    k=0;
end

t=t+Ts;

if t<=0.02
    if u>0.5
        k=0.5;
    else
        k=u;
    end
elseif t>0.02
    k=0.5;
end
    y=k;
